simulink subsystem "VehicleBody1DOFLongitudinal"  (R2023b)
settings: Solver=VariableStepAuto  StartTime=0.0  StopTime=10.0  RelTol=1e-3
undefined symbols (not defined in the file): EnvAirTemp, EnvGrvty, PlntVehCGHgtAxl, PlntVehDstCGRearAxl, PlntVehHtchDst, PlntVehHtchHgtAxl, PlntVehHtchLatDst, PlntVehMass
libraries: autolibshared x1
settings Model: ModifiedByFormat=The MathWorks, Inc.  Creator=The MathWorks, Inc.  LastModifiedBy=The MathWorks, Inc.
settings OptimizationCC: ReuseModelBlockBuffer=off
settings DebuggingCC: SubsystemReferenceDiagnosticForUnitTest=warning

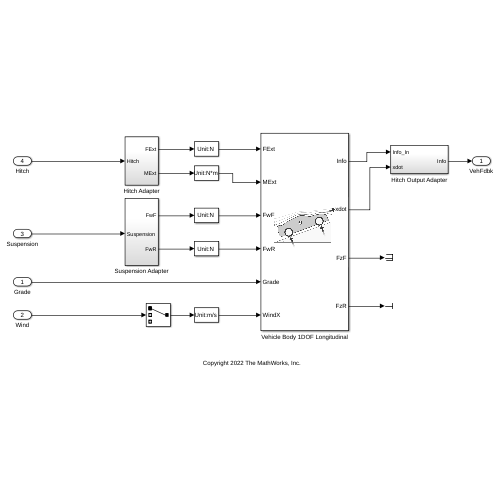
[thumbnail: Simulink's stored preview of the top-level diagram]
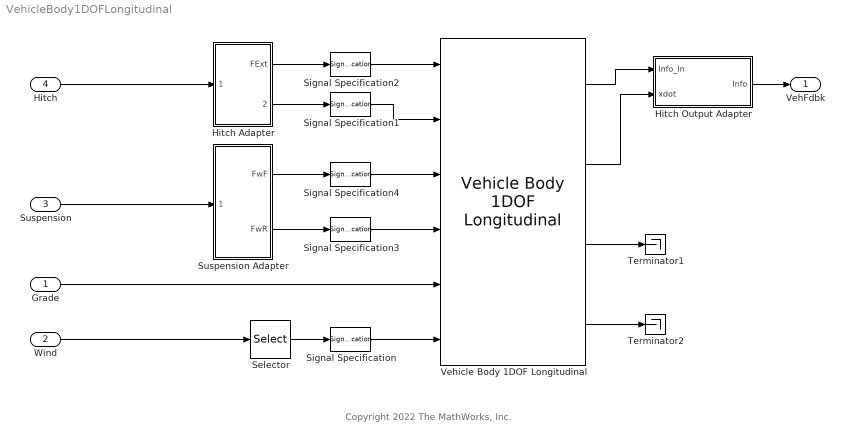
== system VehicleBody1DOFLongitudinal ==
  note: Copyright 2022 The MathWorks, Inc.
  Grade : Inport  Unit=deg
  Wind : Inport  Port=2  Unit=m/s
  Suspension : Inport  Port=3
  Hitch : Inport  Port=4
  Hitch Adapter : Subsystem
  Hitch Output Adapter : Subsystem
  Selector : Selector  InputPortWidth=3  IndexOptions=Index vector (dialog)  Indices=[1]  OutputSizes=1
  Signal Specification : SignalSpecification  Unit=m/s
  Signal Specification1 : SignalSpecification  Unit=N*m
  Signal Specification2 : SignalSpecification  Unit=N
  Signal Specification3 : SignalSpecification  Unit=N
  Signal Specification4 : SignalSpecification  Unit=N
  Suspension Adapter : Subsystem
  Terminator1 : Terminator
  Terminator2 : Terminator
  Vehicle Body 1DOF Longitudinal : autolibshared/Vehicle Body 1DOF Longitudinal  VariantControl=SL  extFMode=on  extMMode=on  extTamb=off  wind3D=off  aMode=6  NF=PlntVehNumWhlFrntAxl  NR=PlntVehNumWhlRearAxl  m=PlntVehMass  a=PlntVehDstCGFrntAxl  b=PlntVehDstCGRearAxl  h=PlntVehCGHgtAxl  Cd=PlntVehAeroDragCff  Cl=PlntVehAeroLiftCff  Cpm=PlntVehAeroPitchCff  Af=PlntVehAeroFrntArea  x_o=PlntVehInitLongPos  xdot_o=PlntVehInitLongVel  Pabs=EnvAbsPrs  T=EnvAirTemp  g=EnvGrvty
  VehFdbk : Outport  VectorParamsAs1DForOutWhenUnconnected=off
  wires:
  Wind/1 -> Selector/1
  Selector/1 -> Signal Specification/1
  Signal Specification4/1 -> Vehicle Body 1DOF Longitudinal/3
  Signal Specification3/1 -> Vehicle Body 1DOF Longitudinal/4
  Grade/1 -> Vehicle Body 1DOF Longitudinal/5
  Signal Specification/1 -> Vehicle Body 1DOF Longitudinal/6
  Vehicle Body 1DOF Longitudinal/1 -> Hitch Output Adapter/1(Info_In)
  Hitch Output Adapter/1(Info) -> VehFdbk/1
  Vehicle Body 1DOF Longitudinal/2 -> Hitch Output Adapter/2(xdot)
  Vehicle Body 1DOF Longitudinal/3 -> Terminator1/1
  Vehicle Body 1DOF Longitudinal/4 -> Terminator2/1
  Suspension/1 -> Suspension Adapter/1(Suspension)
  Suspension Adapter/1(FwF) -> Signal Specification4/1
  Suspension Adapter/2(FwR) -> Signal Specification3/1
  Hitch Adapter/2(MExt) -> Signal Specification1/1
  Hitch/1 -> Hitch Adapter/1(Hitch)
  Hitch Adapter/1(FExt) -> Signal Specification2/1
  Signal Specification1/1 -> Vehicle Body 1DOF Longitudinal/2
  Signal Specification2/1 -> Vehicle Body 1DOF Longitudinal/1

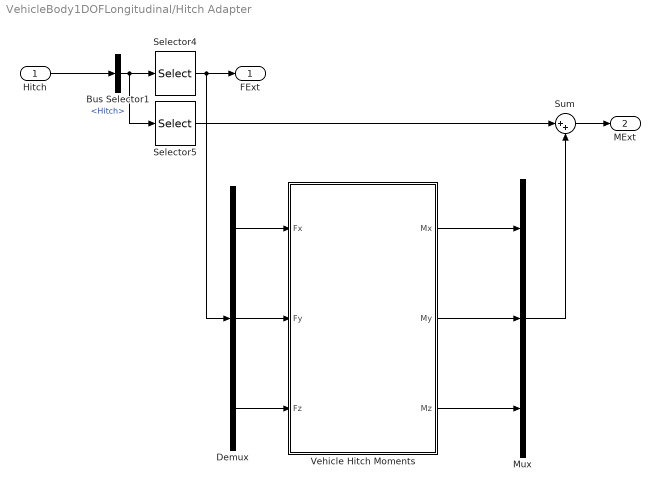
== system VehicleBody1DOFLongitudinal/Hitch Adapter ==
  Hitch : Inport
  Bus Selector1 : BusSelector  OutputSignals=Hitch
  Demux : Demux  Outputs=3
  Mux : Mux  Inputs=3
  Selector4 : Selector  InputPortWidth=6  IndexOptions=Index vector (dialog)  Indices=[1:3]  OutputSizes=1
  Selector5 : Selector  InputPortWidth=6  IndexOptions=Index vector (dialog)  Indices=[4:6]  OutputSizes=1
  Sum : Sum  Inputs=|++
  Vehicle Hitch Moments : Subsystem  mask{h=PlntVehCGHgtAxl, dh=PlntVehHtchDst, hh=PlntVehHtchHgtAxl, hl=PlntVehHtchLatDst}
      mask prompts: h "vdynblks:vehdynTractorBody6Dof:blkPrm_h"; dh "vdynblks:vehdynTractorBody6Dof:blkPrm_dh"; hh "vdynblks:vehdynTractorBody6Dof:blkPrm_hh"; hl "vdynblks:vehdynTractorBody6Dof:blkPrm_hl"
      mask DialogControl h Prompt: Vertical distance from center of mass to axle plane, h [m]:
      mask DialogControl dh Prompt: Longitudinal distance from center of mass to hitch, dh [m]:
      mask DialogControl hh Prompt: Vertical distance from hitch to axle plane, hh [m]:
      mask DialogControl hl Prompt: Lateral distance from geometric centerline to hitch, hl [m]:
  FExt : Outport
  MExt : Outport  Port=2
  wires:
  Selector5/1 -> Sum/1
  Bus Selector1/1 -> Selector5/1, Selector4/1  "<Hitch>"
  Selector4/1 -> FExt/1, Demux/1
  Hitch/1 -> Bus Selector1/1
  Demux/1 -> Vehicle Hitch Moments/1(Fx)
  Demux/2 -> Vehicle Hitch Moments/2(Fy)
  Demux/3 -> Vehicle Hitch Moments/3(Fz)
  Vehicle Hitch Moments/1(Mx) -> Mux/1
  Vehicle Hitch Moments/2(My) -> Mux/2
  Vehicle Hitch Moments/3(Mz) -> Mux/3
  Sum/1 -> MExt/1
  Mux/1 -> Sum/2

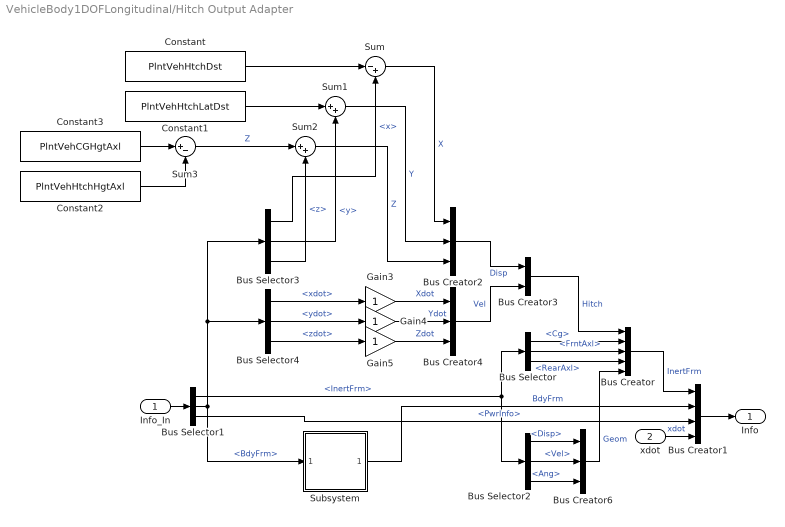
== system VehicleBody1DOFLongitudinal/Hitch Output Adapter ==
  Info_In : Inport
  xdot : Inport  Port=2
  Bus Creator : BusCreator  Inputs=5
  Bus Creator1 : BusCreator  Inputs=4
  Bus Creator2 : BusCreator  Inputs=3
  Bus Creator3 : BusCreator  Inputs=2
  Bus Creator4 : BusCreator  Inputs=3
  Bus Creator6 : BusCreator  Inputs=3
  Bus Selector : BusSelector  OutputSignals=Cg,FrntAxl,RearAxl
  Bus Selector1 : BusSelector  OutputSignals=InertFrm,BdyFrm,PwrInfo
  Bus Selector2 : BusSelector  OutputSignals=Cg.Disp,Cg.Vel,Cg.Ang
  Bus Selector3 : BusSelector  OutputSignals=Cg.Disp.x,Cg.Disp.y,Cg.Disp.z
  Bus Selector4 : BusSelector  OutputSignals=Cg.Vel.xdot,Cg.Vel.ydot,Cg.Vel.zdot
  Constant : Constant  Value=PlntVehHtchDst  SampleTime=-1
  Constant1 : Constant  Value=PlntVehHtchLatDst  SampleTime=-1
  Constant2 : Constant  Value=PlntVehHtchHgtAxl  SampleTime=-1
  Constant3 : Constant  Value=PlntVehCGHgtAxl  SampleTime=-1
  Gain3 : Gain
  Gain4 : Gain
  Gain5 : Gain
  Subsystem : Subsystem
  Sum : Sum  Inputs=|-+
  Sum1 : Sum  Inputs=|++
  Sum2 : Sum  Inputs=|++
  Sum3 : Sum  Inputs=|+-
  Info : Outport
  wires:
  xdot/1 -> Bus Creator1/4  "xdot"
  Subsystem/1(Outport) -> Bus Creator1/2  "BdyFrm"
  Bus Selector2/3 -> Bus Creator6/3  "<Ang>"
  Bus Selector2/2 -> Bus Creator6/2  "<Vel>"
  Bus Selector2/1 -> Bus Creator6/1  "<Disp>"
  Bus Creator6/1 -> Bus Creator/5  "Geom"
  Bus Selector1/2 -> Bus Selector4/1, Bus Selector3/1, Subsystem/1(Inport)  "<BdyFrm>"
  Info_In/1 -> Bus Selector1/1
  Bus Creator/1 -> Bus Creator1/1  "InertFrm"
  Bus Selector3/3 -> Sum2/2  "<z>"
  Bus Selector/3 -> Bus Creator/4  "<RearAxl>"
  Bus Selector1/1 -> Bus Selector/1, Bus Selector2/1  "<InertFrm>"
  Bus Creator1/1 -> Info/1
  Bus Creator3/1 -> Bus Creator/1  "Hitch"
  Bus Selector1/3 -> Bus Creator1/3  "<PwrInfo>"
  Bus Selector3/1 -> Sum/2  "<x>"
  Bus Selector/1 -> Bus Creator/2  "<Cg>"
  Bus Selector/2 -> Bus Creator/3  "<FrntAxl>"
  Bus Creator4/1 -> Bus Creator3/2  "Vel"
  Bus Selector3/2 -> Sum1/2  "<y>"
  Bus Creator2/1 -> Bus Creator3/1  "Disp"
  Bus Selector4/1 -> Gain3/1  "<xdot>"
  Bus Selector4/2 -> Gain4/1  "<ydot>"
  Bus Selector4/3 -> Gain5/1  "<zdot>"
  Gain3/1 -> Bus Creator4/1  "Xdot"
  Gain4/1 -> Bus Creator4/2  "Ydot"
  Gain5/1 -> Bus Creator4/3  "Zdot"
  Constant/1 -> Sum/1
  Sum3/1 -> Sum2/1  "Z"
  Constant3/1 -> Sum3/1
  Sum2/1 -> Bus Creator2/3  "Z"
  Constant2/1 -> Sum3/2
  Sum/1 -> Bus Creator2/1  "X"
  Sum1/1 -> Bus Creator2/2  "Y"
  Constant1/1 -> Sum1/1

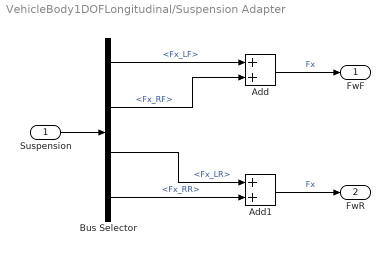
== system VehicleBody1DOFLongitudinal/Suspension Adapter ==
  Suspension : Inport
  Add : Sum
  Add1 : Sum
  Bus Selector : BusSelector  OutputSignals=SuspWheel.Wheels.Fx.Fx_LF,SuspWheel.Wheels.Fx.Fx_RF,SuspWheel.Wheels.Fx.Fx_LR,SuspWheel.Wheels.Fx.Fx_RR
  FwF : Outport
  FwR : Outport  Port=2
  wires:
  Bus Selector/4 -> Add1/2  "<Fx_RR>"
  Bus Selector/3 -> Add1/1  "<Fx_LR>"
  Bus Selector/2 -> Add/2  "<Fx_RF>"
  Bus Selector/1 -> Add/1  "<Fx_LF>"
  Add/1 -> FwF/1  "Fx"
  Add1/1 -> FwR/1  "Fx"
  Suspension/1 -> Bus Selector/1

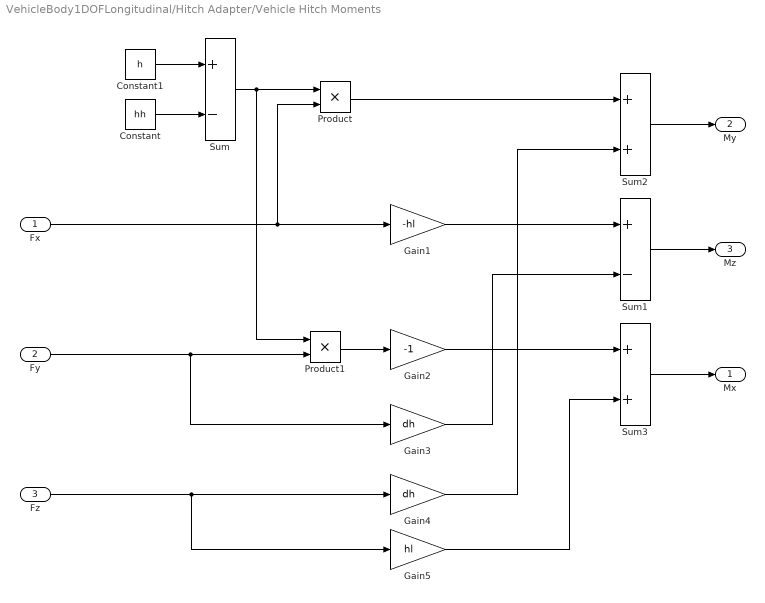
== system VehicleBody1DOFLongitudinal/Hitch Adapter/Vehicle Hitch Moments ==
  Fx : Inport
  Fy : Inport  Port=2
  Fz : Inport  Port=3
  Constant : Constant  Value=hh  SampleTime=-1
  Constant1 : Constant  Value=h  SampleTime=-1
  Gain1 : Gain  Gain=-hl
  Gain2 : Gain  Gain=-1
  Gain3 : Gain  Gain=dh
  Gain4 : Gain  Gain=dh
  Gain5 : Gain  Gain=hl
  Product : Product
  Product1 : Product
  Sum : Sum  Inputs=+-
  Sum1 : Sum  Inputs=+-
  Sum2 : Sum
  Sum3 : Sum
  Mx : Outport
  My : Outport  Port=2
  Mz : Outport  Port=3
  wires:
  Fy/1 -> Gain3/1, Product1/2
  Product1/1 -> Gain2/1
  Sum/1 -> Product1/1, Product/1
  Product/1 -> Sum2/1
  Constant1/1 -> Sum/1
  Gain3/1 -> Sum1/2
  Fx/1 -> Product/2, Gain1/1
  Fz/1 -> Gain5/1, Gain4/1
  Sum2/1 -> My/1
  Constant/1 -> Sum/2
  Gain1/1 -> Sum1/1
  Gain4/1 -> Sum2/2
  Gain5/1 -> Sum3/2
  Gain2/1 -> Sum3/1
  Sum1/1 -> Mz/1
  Sum3/1 -> Mx/1

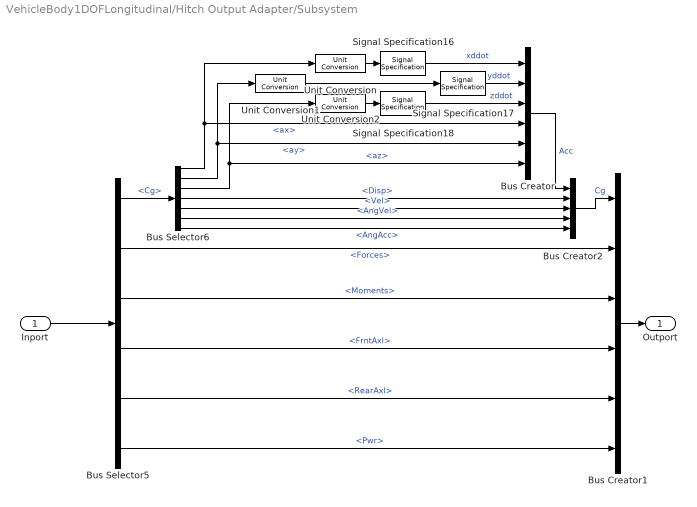
== system VehicleBody1DOFLongitudinal/Hitch Output Adapter/Subsystem ==
  Inport : Inport
  Bus Creator : BusCreator  Inputs=6
  Bus Creator1 : BusCreator  Inputs=6
  Bus Creator2 : BusCreator  Inputs=5
  Bus Selector5 : BusSelector  OutputSignals=Cg,Forces,Moments,FrntAxl,RearAxl,Pwr
  Bus Selector6 : BusSelector  OutputSignals=Acc.ax,Acc.ay,Acc.az,Disp,Vel,AngVel,AngAcc
  Signal Specification16 : SignalSpecification  Unit=m/s^2
  Signal Specification17 : SignalSpecification  Unit=m/s^2
  Signal Specification18 : SignalSpecification  Unit=m/s^2
  Unit Conversion : UnitConversion
  Unit Conversion1 : UnitConversion
  Unit Conversion2 : UnitConversion
  Outport : Outport
  wires:
  Unit Conversion2/1 -> Signal Specification18/1
  Unit Conversion1/1 -> Signal Specification17/1
  Unit Conversion/1 -> Signal Specification16/1
  Bus Creator2/1 -> Bus Creator1/1  "Cg"
  Bus Selector6/6 -> Bus Creator2/4  "<AngVel>"
  Bus Selector6/7 -> Bus Creator2/5  "<AngAcc>"
  Bus Selector6/5 -> Bus Creator2/3  "<Vel>"
  Bus Selector6/4 -> Bus Creator2/2  "<Disp>"
  Bus Creator1/1 -> Outport/1
  Bus Selector5/6 -> Bus Creator1/6  "<Pwr>"
  Bus Selector5/5 -> Bus Creator1/5  "<RearAxl>"
  Bus Selector5/4 -> Bus Creator1/4  "<FrntAxl>"
  Bus Selector5/3 -> Bus Creator1/3  "<Moments>"
  Bus Selector5/2 -> Bus Creator1/2  "<Forces>"
  Bus Creator/1 -> Bus Creator2/1  "Acc"
  Bus Selector6/3 -> Bus Creator/6, Unit Conversion2/1  "<az>"
  Inport/1 -> Bus Selector5/1
  Signal Specification18/1 -> Bus Creator/3  "zddot"
  Signal Specification16/1 -> Bus Creator/1  "xddot"
  Signal Specification17/1 -> Bus Creator/2  "yddot"
  Bus Selector6/1 -> Unit Conversion/1, Bus Creator/4  "<ax>"
  Bus Selector6/2 -> Unit Conversion1/1, Bus Creator/5  "<ay>"
  Bus Selector5/1 -> Bus Selector6/1  "<Cg>"
